simulink subsystem "TractionControll"  (R2021b)
settings: Solver=VariableStepAuto  StartTime=0.0  StopTime=10.0  RelTol=1e-3
undefined symbols (not defined in the file): DiscIntNeverNeededParam
libraries: simulink x2
settings Model: Creator=tsuyoshi  LastModifiedBy=tsuyoshi

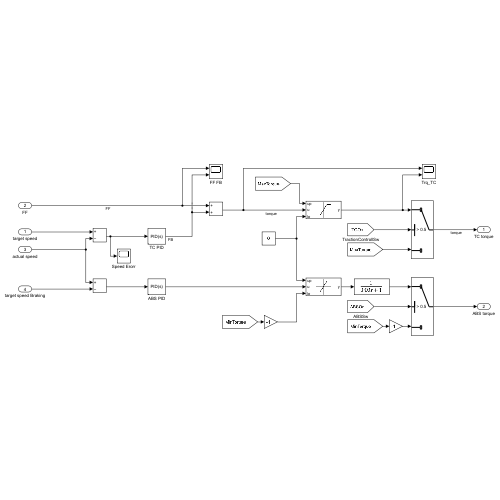
[thumbnail: Simulink's stored preview of the top-level diagram]
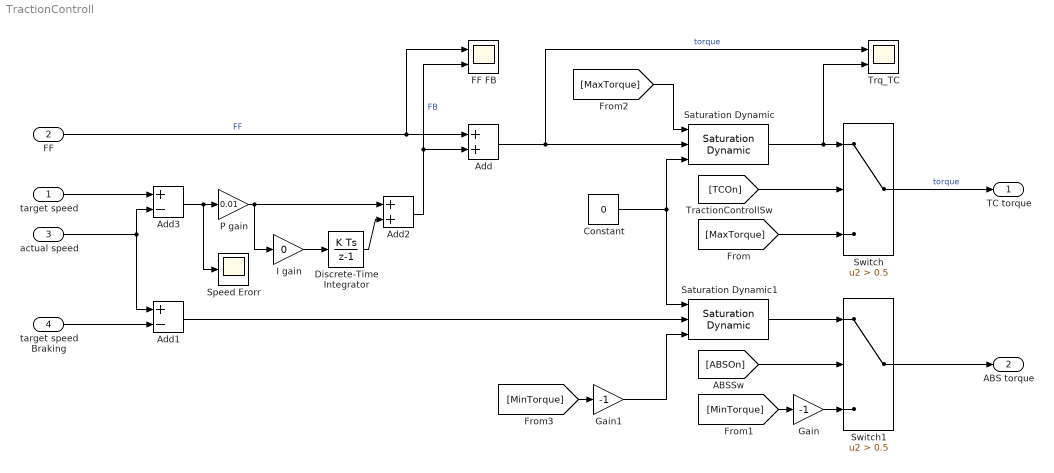
== system TractionControll ==
  target speed : Inport
  FF : Inport  Port=2
  actual speed : Inport  Port=3
  target speed Braking : Inport  Port=4
  Add : Sum
  Add1 : Sum  Inputs=+-
  Add2 : Sum
  Add3 : Sum  Inputs=+-
  Constant : Constant  Value=0
  Discrete-Time Integrator : DiscreteIntegrator  gainval=1  SampleTime=-1  ICPrevOutput=DiscIntNeverNeededParam  ICPrevScaledInput=DiscIntNeverNeededParam
  FF FB : Scope  NumInputPorts=2
  Gain : Gain  Gain=-1
  Gain1 : Gain  Gain=-1
  I gain : Gain  Gain=0
  P gain : Gain  Gain=0.01
  Saturation Dynamic : simulink/Discontinuities/Saturation Dynamic  OutMin=[]  OutMax=[]  OutDataTypeStr=Inherit: Same as second input  OutDataType=fixdt(1, 16)  OutScaling=2^-10  DoSatur=off
  Saturation Dynamic1 : simulink/Discontinuities/Saturation Dynamic  OutMin=[]  OutMax=[]  OutDataTypeStr=Inherit: Same as second input  OutDataType=fixdt(1, 16)  OutScaling=2^-10  DoSatur=off
  Speed Erorr : Scope
  Switch : Switch  Criteria=u2 > Threshold  Threshold=0.5
  Switch1 : Switch  Criteria=u2 > Threshold  Threshold=0.5
  Trq_TC : Scope  NumInputPorts=2
  TC torque : Outport  VectorParamsAs1DForOutWhenUnconnected=off
  ABS torque : Outport  Port=2  VectorParamsAs1DForOutWhenUnconnected=off
  wires:
  I gain/1 -> Discrete-Time Integrator/1
  Saturation Dynamic1/1 -> Switch1/1
  Gain1/1 -> Saturation Dynamic1/3
  [MinTorque] -> Gain1/1
  Add1/1 -> Saturation Dynamic1/2
  Constant/1 -> Saturation Dynamic1/1, Saturation Dynamic/3
  [MaxTorque] -> Saturation Dynamic/1
  [MinTorque] -> Gain/1
  Switch1/1 -> ABS torque/1
  [ABSOn] -> Switch1/2
  Gain/1 -> Switch1/3
  [MaxTorque] -> Switch/3
  [TCOn] -> Switch/2
  target speed Braking/1 -> Add1/2
  Add3/1 -> Speed Erorr/1, P gain/1
  target speed/1 -> Add3/1
  actual speed/1 -> Add3/2, Add1/1
  Add/1 -> Saturation Dynamic/2, Trq_TC/1  "torque"
  Switch/1 -> TC torque/1  "torque"
  Add2/1 -> Add/2, FF FB/2  "FB"
  Saturation Dynamic/1 -> Switch/1, Trq_TC/2
  FF/1 -> FF FB/1, Add/1  "FF"
  Discrete-Time Integrator/1 -> Add2/2
  P gain/1 -> I gain/1, Add2/1
